simulink model "auv_6dof_sim"  (R2015b)
settings: Solver=VariableStepAuto  StartTime=0.0  StopTime=10.0  RelTol=1e-3
libraries: simulink x6
settings Model: Creator=drew  LastModifiedBy=drew

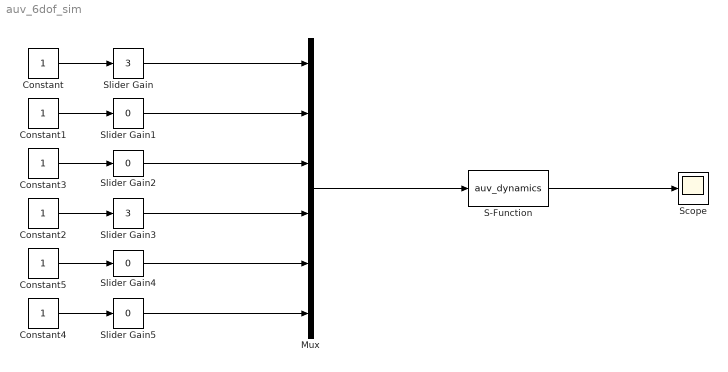
== system auv_6dof_sim ==
  Constant{,1..5} (6 alike) : Constant
  Mux : Mux  Inputs=6
  S-Function : S-Function  FunctionName=auv_dynamics  Parameters=P  SFunctionDeploymentMode=off  EnableBusSupport=off
  Scope : Scope
  Slider Gain : simulink/Math Operations/Slider Gain  low=-50  gain=3  high=50
  Slider Gain{1..2,4..5} (4 alike) : simulink/Math Operations/Slider Gain  low=-50  gain=0  high=50
  Slider Gain3 : simulink/Math Operations/Slider Gain  low=-50  gain=3  high=50
  wires:
  Constant/1 -> Slider Gain/1
  Constant3/1 -> Slider Gain2/1
  Constant1/1 -> Slider Gain1/1
  Constant2/1 -> Slider Gain3/1
  Constant4/1 -> Slider Gain5/1
  Constant5/1 -> Slider Gain4/1
  Slider Gain/1 -> Mux/1
  Slider Gain1/1 -> Mux/2
  Slider Gain2/1 -> Mux/3
  Slider Gain3/1 -> Mux/4
  Slider Gain4/1 -> Mux/5
  Slider Gain5/1 -> Mux/6
  Mux/1 -> S-Function/1
  S-Function/1 -> Scope/1
